simulink model "miniprojekt_sim"  (R2018a)
settings: Solver=VariableStepAuto  StartTime=0.0  StopTime=10000  RelTol=1e-3
values from neighbouring files (symbols this model uses):
  cp = 1005    [miniprojekt.m]
  cvp = cp*rop*Vp    (= 241200)    [miniprojekt.m]
  cvw = cp*rop*Vw    (= 3618000)    [miniprojekt.m]
  fp = 1    [miniprojekt.m]
  k1 = x(1,1)    [miniprojekt.m]    (also in miniprojekt_2.m)
  kp = 1/4*kw    [miniprojekt.m]    (also in miniprojekt_2.m = mnoznik*kw)
  kw = x(2,1)    [miniprojekt.m]    (also in miniprojekt_2.m)
  rop = 1.2    [miniprojekt.m]
  Tp0 = Tp    (= 18)    [miniprojekt.m]    (also in miniprojekt_2.m = Tp05)
  Twew0 = Twew    (= 24)    [miniprojekt.m]    (also in miniprojekt_2.m = Twew05)
  Tz = 26    [miniprojekt.m]
  Tzew = 26    [miniprojekt.m]
settings Model: Creator=jacek  LastModifiedBy=johnb
settings DataIOCC: ReturnWorkspaceOutputs=on
settings SFSimCC: SimUseLocalCustomCode=on
settings RTWCC: RTWUseLocalCustomCode=on

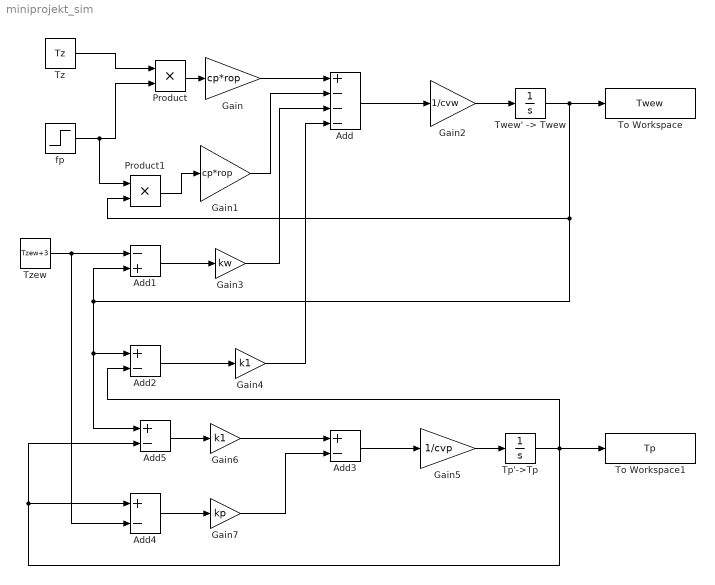
== system miniprojekt_sim ==
  Add : Sum  Inputs=+---
  Add1 : Sum  Inputs=-+
  Add{2..5} (4 alike) : Sum  Inputs=+-
  Gain : Gain  Gain=cp*rop
  Gain1 : Gain  Gain=cp*rop
  Gain2 : Gain  Gain=1/cvw
  Gain3 : Gain  Gain=kw
  Gain4 : Gain  Gain=k1
  Gain5 : Gain  Gain=1/cvp
  Gain6 : Gain  Gain=k1
  Gain7 : Gain  Gain=kp
  Product : Product
  Product1 : Product
  To Workspace : ToWorkspace  VariableName=Twew  SampleTime=-1
  To Workspace1 : ToWorkspace  VariableName=Tp  SampleTime=-1
  Tp'->Tp : Integrator  InitialCondition=Tp0
  "Twew' -> Twew" : Integrator  InitialCondition=Twew0
  Tz : Constant  Value=Tz
  Tzew : Constant  Value=Tzew+3
  fp : Step  Before=fp  After=fp  SampleTime=0
  wires:
  Tz/1 -> Product/1
  fp/1 -> Product1/1, Product/2
  Product/1 -> Gain/1
  Gain2/1 -> "Twew' -> Twew"/1
  Gain/1 -> Add/1
  Product1/1 -> Gain1/1
  Gain1/1 -> Add/2
  Add1/1 -> Gain3/1
  Gain3/1 -> Add/3
  Add2/1 -> Gain4/1
  Gain4/1 -> Add/4
  Add/1 -> Gain2/1
  "Twew' -> Twew"/1 -> To Workspace/1, Add5/1, Add2/1, Add1/2, Product1/2
  Tzew/1 -> Add4/2, Add1/1
  Gain5/1 -> Tp'->Tp/1
  Add3/1 -> Gain5/1
  Gain6/1 -> Add3/1
  Gain7/1 -> Add3/2
  Add5/1 -> Gain6/1
  Add4/1 -> Gain7/1
  Tp'->Tp/1 -> To Workspace1/1, Add2/2, Add4/1, Add5/2
